simulink model "General_AC_Machine"  (R2020a)
settings: Solver=ode45  StartTime=0.0  StopTime=10.0  RelTol=1e-3  EnableMultiTasking=on
values from neighbouring files (symbols this model uses):
  L_m = 0.326    [Experiment_3_ASM_Parameter.m]
  L_r = 0.340    (= 0.34)    [Experiment_3_ASM_Parameter.m]
  L_s = 0.340    (= 0.34)    [Experiment_3_ASM_Parameter.m]    (also in Experiment_3_PMSM_Parameter.m = 0.012)
  L_sigma_r = L_r - L_m    (= 0.014)    [Experiment_3_ASM_Parameter.m]
  L_sigma_s = L_s - L_m    (= 0.014)    [Experiment_3_ASM_Parameter.m]
  p = 1    [Experiment_3_ASM_Parameter.m]    (also in Experiment_3_PMSM_Parameter.m = 3)
  R_r = 2.9    [Experiment_3_ASM_Parameter.m]
  R_s = 2.2    [Experiment_3_ASM_Parameter.m]    (also in Experiment_3_PMSM_Parameter.m = 1.2)
  sigma = (L_s*L_r - L_m^2)/(L_s*L_r)    (= 0.0806574394464)    [Experiment_3_ASM_Parameter.m]
  Theta_M = 0.02    [Experiment_3_ASM_Parameter.m]    (also in Experiment_3_PMSM_Parameter.m = 0.001)
settings Model: Creator=julien  LastModifiedBy=ge29wel
settings DataIOCC: LimitDataPoints=on  SaveFormat=Array  ReturnWorkspaceOutputs=off
settings OptimizationCC: ExpressionDepthLimit=2147483647  LifeSpan=inf
settings DebuggingCC: UnderspecifiedInitializationDetection=Classic  MergeDetectMultiDrivingBlocksExec=none  SolverPrmCheckMsg=warning  StateNameClashWarn=warning  SFUnexpectedBacktrackingDiag=warning  SFNoUnconditionalDefaultTransitionDiag=warning  SFExecutionAtInitializationDiag=none  ArithmeticOperatorsInVariantConditions=warning
settings HardwareCC: ProdBitPerPointer=32  ProdBitPerSizeT=32  ProdBitPerPtrDiffT=32  ProdLargestAtomicFloat=None  ProdIntDivRoundTo=Undefined  ProdEndianess=Unspecified  ProdWordSize=32  ProdHWDeviceType=32-bit Generic
settings ModelReferenceCC: PropagateSignalLabelsOutOfModel=off
settings SFSimCC: SimUseLocalCustomCode=off  CustomCodeUndefinedFunction=UseInterfaceOnly
settings RTWCC: RTWUseLocalCustomCode=off
settings CodeAppCC: StateflowObjectComments=on
settings GRTTargetCC: TargetLangStandard=C89/C90 (ANSI)
settings ConfigComp: CovMetricSettings=dw  CovHtmlReporting=on  CovSaveCumulativeToWorkspaceVar=on  CovSaveSingleToWorkspaceVar=on  CovExternalEMLEnable=off  CovSFcnEnable=off

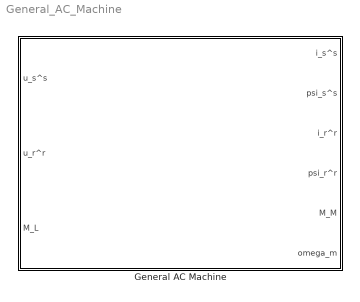
== system General_AC_Machine ==
  General AC Machine : Subsystem

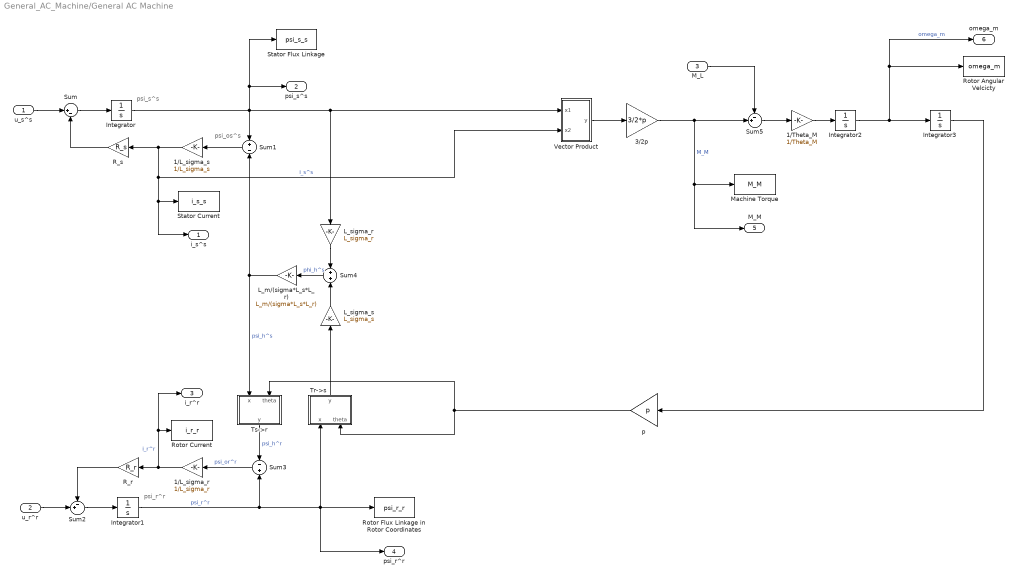
== system General_AC_Machine/General AC Machine ==
  note: psi_s^s
  note: psi_r^r
  note: psi_os^s
  u_s^s : Inport
  u_r^r : Inport  Port=2
  M_L : Inport  Port=3
  1/L_sigma_r : Gain  Gain=1/L_sigma_r
  1/L_sigma_s : Gain  Gain=1/L_sigma_s
  1/Theta_M : Gain  Gain=1/Theta_M
  3/2p : Gain  Gain=3/2*p
  Integrator{,1..3} (4 alike) : Integrator
  L_m/(sigma*L_s*L_r) : Gain  Gain=L_m/(sigma*L_s*L_r)
  L_sigma_r : Gain  Gain=L_sigma_r
  L_sigma_s : Gain  Gain=L_sigma_s
  Machine Torque : ToWorkspace  VariableName=M_M  SaveFormat=Timeseries  SampleTime=-1
  R_r : Gain  Gain=R_r
  R_s : Gain  Gain=R_s
  Rotor Angular Velcicty : ToWorkspace  VariableName=omega_m  SaveFormat=Timeseries  SampleTime=-1
  Rotor Current : ToWorkspace  VariableName=i_r_r  SaveFormat=Timeseries  SampleTime=-1
  Rotor Flux Linkage in Rotor Coordinates : ToWorkspace  VariableName=psi_r_r  SaveFormat=Timeseries  SampleTime=-1
  Stator Current : ToWorkspace  VariableName=i_s_s  SaveFormat=Timeseries  SampleTime=-1
  Stator Flux Linkage : ToWorkspace  VariableName=psi_s_s  SaveFormat=Timeseries  SampleTime=-1
  Sum : Sum  Inputs=|+-
  Sum1 : Sum  Inputs=+|-
  Sum2 : Sum  Inputs=-+|
  Sum3 : Sum  Inputs=-|+
  Sum4 : Sum  Inputs=+|+
  Sum5 : Sum  Inputs=-+|
  Tr->s : Subsystem
  Ts->r : Subsystem
  Vector Product : Subsystem
  p : Gain  Gain=p
  i_s^s : Outport
  psi_s^s : Outport  Port=2
  i_r^r : Outport  Port=3
  psi_r^r : Outport  Port=4
  M_M : Outport  Port=5
  omega_m : Outport  Port=6
  wires:
  u_s^s/1 -> Sum/1
  R_s/1 -> Sum/2
  Sum/1 -> Integrator/1
  1/L_sigma_s/1 -> R_s/1, Stator Current/1, i_s^s/1, Vector Product/2(x2)  "i_s^s"
  Integrator/1 -> psi_s^s/1, Stator Flux Linkage/1, Sum1/1, L_sigma_r/1, Vector Product/1(x1)
  Sum1/1 -> 1/L_sigma_s/1
  u_r^r/1 -> Sum2/2
  Sum2/1 -> Integrator1/1
  R_r/1 -> Sum2/1
  1/L_sigma_r/1 -> R_r/1, Rotor Current/1, i_r^r/1  "i_r^r"
  Integrator1/1 -> Sum3/2, psi_r^r/1, Tr->s/1(x), Rotor Flux Linkage in Rotor Coordinates/1  "psi_r^r"
  Sum3/1 -> 1/L_sigma_r/1  "psi_or^r"
  Tr->s/1(y) -> L_sigma_s/1
  L_sigma_r/1 -> Sum4/1
  L_sigma_s/1 -> Sum4/2
  Vector Product/1(y) -> 3/2p/1
  3/2p/1 -> Machine Torque/1, M_M/1, Sum5/2  "M_M"
  M_L/1 -> Sum5/1
  Sum5/1 -> 1/Theta_M/1
  1/Theta_M/1 -> Integrator2/1
  Integrator2/1 -> Integrator3/1, Rotor Angular Velcicty/1, omega_m/1  "omega_m"
  Integrator3/1 -> p/1
  Ts->r/1(y) -> Sum3/1  "psi_h^r"
  L_m/(sigma*L_s*L_r)/1 -> Sum1/2, Ts->r/1(x)  "psi_h^s"
  p/1 -> Ts->r/2(theta), Tr->s/2(theta)
  Sum4/1 -> L_m/(sigma*L_s*L_r)/1  "phi_h^s"

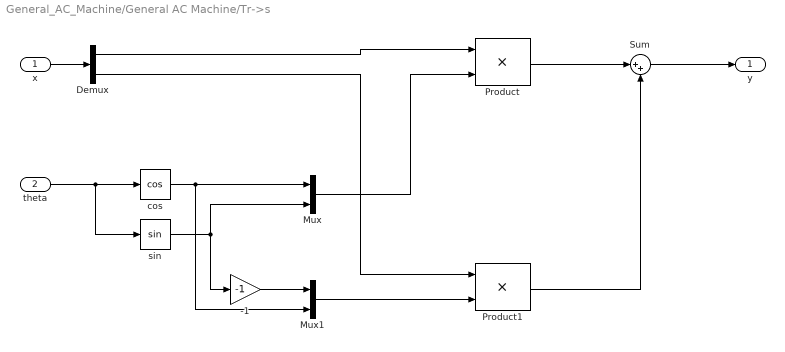
== system General_AC_Machine/General AC Machine/Tr->s ==
  x : Inport
  theta : Inport  Port=2
  -1 : Gain  Gain=-1
  Demux : Demux  Outputs=2
  Mux : Mux  Inputs=2
  Mux1 : Mux  Inputs=2
  Product : Product  RndMeth=Zero
  Product1 : Product  RndMeth=Zero
  Sum : Sum  Inputs=|++
  cos : Trigonometry  Operator=cos
  sin : Trigonometry
  y : Outport
  wires:
  x/1 -> Demux/1
  theta/1 -> cos/1, sin/1
  cos/1 -> Mux/1, Mux1/2
  sin/1 -> Mux/2, -1/1
  Mux/1 -> Product/2
  -1/1 -> Mux1/1
  Mux1/1 -> Product1/2
  Demux/2 -> Product1/1
  Product/1 -> Sum/1
  Product1/1 -> Sum/2
  Sum/1 -> y/1
  Demux/1 -> Product/1

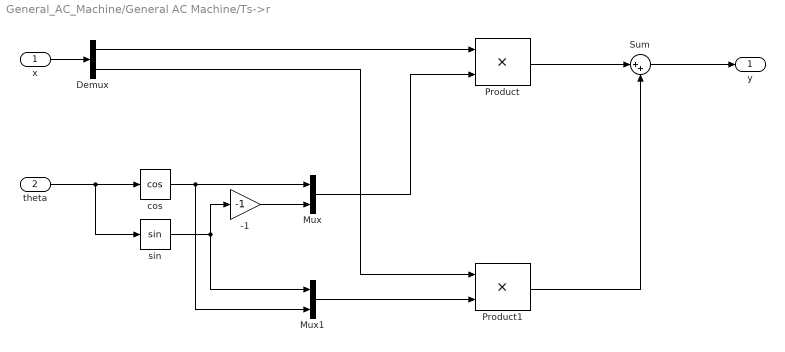
== system General_AC_Machine/General AC Machine/Ts->r ==
  x : Inport
  theta : Inport  Port=2
  -1 : Gain  Gain=-1
  Demux : Demux  Outputs=2
  Mux : Mux  Inputs=2
  Mux1 : Mux  Inputs=2
  Product : Product  RndMeth=Zero
  Product1 : Product  RndMeth=Zero
  Sum : Sum  Inputs=|++
  cos : Trigonometry  Operator=cos
  sin : Trigonometry
  y : Outport
  wires:
  x/1 -> Demux/1
  theta/1 -> cos/1, sin/1
  Demux/1 -> Product/1
  cos/1 -> Mux/1, Mux1/2
  sin/1 -> -1/1, Mux1/1
  Mux/1 -> Product/2
  Mux1/1 -> Product1/2
  Demux/2 -> Product1/1
  Product/1 -> Sum/1
  Product1/1 -> Sum/2
  -1/1 -> Mux/2
  Sum/1 -> y/1

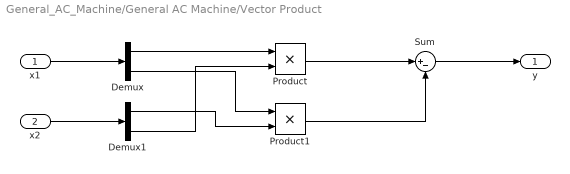
== system General_AC_Machine/General AC Machine/Vector Product ==
  x1 : Inport
  x2 : Inport  Port=2
  Demux : Demux  Outputs=2
  Demux1 : Demux  Outputs=2
  Product : Product  RndMeth=Zero
  Product1 : Product  RndMeth=Zero
  Sum : Sum  Inputs=|+-
  y : Outport
  wires:
  Sum/1 -> y/1
  Product1/1 -> Sum/2
  Product/1 -> Sum/1
  Demux1/1 -> Product1/2
  Demux/2 -> Product1/1
  Demux1/2 -> Product/2
  Demux/1 -> Product/1
  x2/1 -> Demux1/1
  x1/1 -> Demux/1
